simulink subsystem "reaction_wheel_model"  (R2025a)
settings: Solver=VariableStepAuto  StartTime=0.0  StopTime=10.0  RelTol=1e-3
undefined symbols (not defined in the file or in its folder): Actuators, reaction_wheel_state_space_A, reaction_wheel_state_space_B, reaction_wheel_state_space_C, reaction_wheel_state_space_D, reaction_wheel_state_space_initial
settings Model: Creator=joshu  LastModifiedBy=arroy

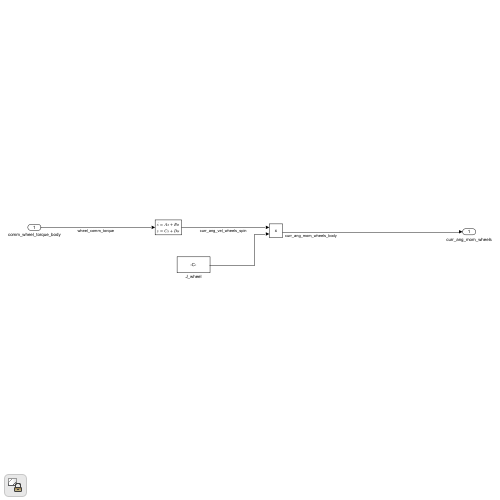
[thumbnail: Simulink's stored preview of the top-level diagram]
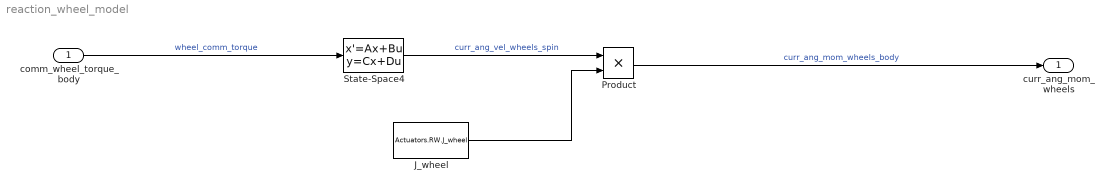
== system reaction_wheel_model ==
  comm_wheel_torque_body : Inport
  J_wheel : Constant  Value=Actuators.RW.J_wheel
  Product : Product
  State-Space4 : StateSpace  A=reaction_wheel_state_space_A  B=reaction_wheel_state_space_B  C=reaction_wheel_state_space_C  D=reaction_wheel_state_space_D  InitialCondition=reaction_wheel_state_space_initial  ParameterTunability=Unconstrained
  curr_ang_mom_wheels : Outport
  wires:
  J_wheel/1 -> Product/2
  State-Space4/1 -> Product/1  "curr_ang_vel_wheels_spin"
  comm_wheel_torque_body/1 -> State-Space4/1  "wheel_comm_torque"
  Product/1 -> curr_ang_mom_wheels/1  "curr_ang_mom_wheels_body"
